simulink model "sf_fxptgf"  (Simulink 7.6)
settings: Solver=ode45  StartTime=0.0  StopTime=13  MaxStep=.1  RelTol=1e-3
settings Model: Creator=The MathWorks Inc.  CovMetricSettings=dcmtr  ExtModeAutoUpdateStatusClock=off
settings DataIOCC: SignalLoggingName=sigsOut
settings OptimizationCC: InlineInvariantSignals=on  InitFltsAndDblsToZero=on  EfficientMapNaN2IntZero=off
settings DebuggingCC: SaveWithParameterizedLinksMsg=none  SignalResolutionControl=TryResolveAllWithWarning  SolverPrmCheckMsg=none  MultiTaskDSMMsg=warning  MultiTaskCondExecSysMsg=none  ParameterOverflowMsg=warning  StrictBusMsg=None
settings HardwareCC: TargetUnknown=on
settings SFSimCC: SimParseCustomCode=off
settings RTWCC: IncludeERTFirstTime=on
settings GRTTargetCC: TargetFcnLib=ansi_tfl_tmw.mat

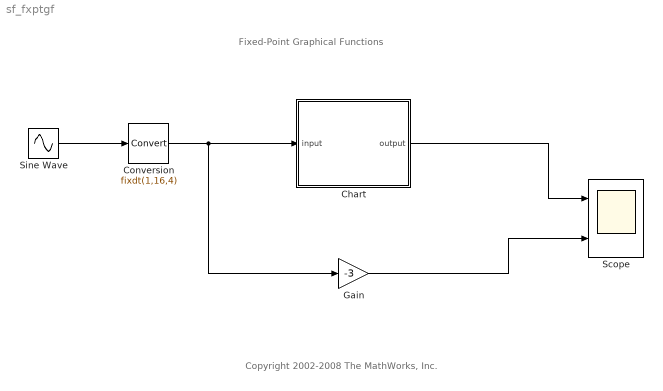
== system sf_fxptgf ==
  note: Fixed-Point Graphical Functions
  note: Copyright 2002-2008 The MathWorks, Inc.
  Chart : Stateflow chart  TreatAsAtomicUnit=on
  Conversion : DataTypeConversion  OutDataTypeStr=fixdt(1,16,4)
  Gain : Gain  Gain=-3  SaturateOnIntegerOverflow=on  OutDataTypeStr=Inherit: Same as input  ParamDataTypeStr=Inherit: Same as input
  Scope : Scope  NumInputPorts=2
      settings: YMin=0~-4  YMax=3~4
  Sine Wave : Sin  SampleTime=0
  wires:
  Sine Wave/1 -> Conversion/1
  Chart/1(output) -> Scope/1
  Gain/1 -> Scope/2
  Conversion/1 -> Chart/1(input), Gain/1

== stateflow chart Chart ==
  state out = fixout(fixin) [function]
    (default) -> (junction 5)
    (junction 5) -> (junction 6) [order 1] : [fixin>=0]{out=3*fixin;}
    (junction 5) -> (junction 7) [order 2] : {out=-3*fixin;}
  (default) -> (junction 4) : {output=fixout(input);}
  data: fixin function_input fixdt(1,16,0.0002,0); out function_output double; input input fixdt(1,16,4); output output double
